simulink model "PubIfDecisionTOS_MDL"  (R2020b)
settings: configuration reference "DspaceConfig" (kept outside this file)
PostLoadFcn:
  | if any(exist('dsrtsu_mdlpostloadfcn', 'file') ~= 0), dsrtsu_mdlpostloadfcn('Execute', bdroot); end
InitFcn:
  | , if any(exist('dsmpb_private', 'file') ~= 0), dsmpb_private('dsmpb_mdlclblib', 'Init', bdroot); end,
undefined symbols (not defined in the file or in its folder): C_TOS_ACCEgoRAxletoFbumplength_m, C_TOS_ACCTargetFront_Flag, C_TOS_AEBJAPedObjDxThre_Val, C_TOS_AEBJAPedObjDyThre_Val, C_TOS_AEBJATargetSize_Val, C_TOS_AEBJAVehObjDxThre_Val, C_TOS_AEBJAVehObjDyThre_Val, C_TOS_AEBJuncPedTargetSize_Val, C_TOS_AEBLatObjDxThre_Val, C_TOS_AEBLatPedDyThre_Val, C_TOS_AEBLatTargetSize_Val, C_TOS_AEBLongTargetInEgoFront_Flag, C_TOS_axAbsGround_Parameter, C_TOS_CameraConfirmedFlag, C_TOS_CNsubjWidth, C_TOS_CurrentLaneCoreMinWidth_Val, C_TOS_CutInProb_Val_Zero, C_TOS_CutOutProb_Val_Zero, C_TOS_D2R_Val, C_TOS_DefaultValueObjectToCenterLine_dy, C_TOS_EgoCarWidth_Val, C_TOS_EgoDxRefPoint_m, C_TOS_EgoRAxletoFbumplength_m, C_TOS_HalfWidthVehicle_Con, C_TOS_HWA_CurrentLaneFlag, C_TOS_HWA_LeftLaneFlag, C_TOS_HWA_MovingDir_Vaild, C_TOS_HWA_MovState_Vaild, C_TOS_HWA_RightLaneFlag, C_TOS_LaneLineCourseErrorFront, C_TOS_LaneLineCourseErrorRear, C_TOS_MotorbikeDefaultWidth_m, C_TOS_NumberOfEffectiveTargets, C_TOS_Obj_Age_Val, C_TOS_Objdx_Constraint_Val, C_TOS_ObjectDefaultWidth_m, C_TOS_ObjInCurrentLane_Val, C_TOS_ObjInCurrentLaneValid, C_TOS_ObjInLeftLaneValid, C_TOS_ObjInRightLaneValid, C_TOS_ObjNotInCurrentLane_Val, C_TOS_ObjNotREElementType, C_TOS_ObjPredictDis_dy_ConstantVal_Zeros, C_TOS_ObjToCenterLine_ConstantVal_Zeros, C_TOS_OFMObjIDInvilad_Val, C_TOS_PIL_LatDisCons_Val_zero, C_TOS_PIL_ObjectCutInFlag_b, C_TOS_PIL_ObjectCutOutFlag_b, C_TOS_PIL_ObjLaneProb_al_Val, C_TOS_PP_ObjFusType_FC_Confirm_b, C_TOS_PP_ObjFusType_FC_FR_Confirm_b, C_TOS_PP_ObjFusType_FR_Confirm_b, C_TOS_RE_80BoolDefault_Val, C_TOS_RE_80Single181Default_Val, C_TOS_RE_80Single255Default_Val, C_TOS_RE_80Uint8Default_Val, C_TOS_RE_D2R, C_TOS_RE_D_180_Val, C_TOS_RE_InvalidObjectID_Val, C_TOS_RE_InvalidTargetChainDir_Val ... (+142)
libraries: simulink x1650, TOS_LIB x361, canfdmsglib x14
(part 12 of 69)

== system PubIfDecisionTOS_MDL/TOS_20201112/TOS_2012080320/TOS/ACC/TOS_ACCLeftLane/ACC_Object_PreConfirm ==
  PP_ObjFusType_FC_FR_Confirm : Inport
  PP_ObjFusType_FR_Confirm : Inport  Port=2
  PP_ObjFusType_FC_Confirm : Inport  Port=3
  Object_ID : Inport  Port=4
  Obj_MovingState : Inport  Port=5
  Obj_Dx : Inport  Port=6
  Object_ObstacleProb : Inport  Port=7
  Object_DY : Inport  Port=8
  Object_Type : Inport  Port=9
  ACC_Target_ID_K1 : Inport  Port=10
  ACC_Target_Dx_K1 : Inport  Port=11
  ACC_Object_PreConfirm : Subsystem
  Bus Creator : BusCreator  Inputs=5
  Unit Delay : UnitDelay  SampleTime=-1  HasFrameUpgradeWarning=on
  Unit Delay1 : UnitDelay  InitialCondition=255  SampleTime=-1  HasFrameUpgradeWarning=on
  TOS_ACC_P2_P4_TargetPreConfirm : Outport
  wires:
  PP_ObjFusType_FR_Confirm/1 -> ACC_Object_PreConfirm/2(PP_ObjFusType_FR_Confirm)
  PP_ObjFusType_FC_FR_Confirm/1 -> ACC_Object_PreConfirm/1(PP_ObjFusType_FC_FR_Confirm)
  PP_ObjFusType_FC_Confirm/1 -> ACC_Object_PreConfirm/3(PP_ObjFusType_FC_Confirm)
  Object_ID/1 -> ACC_Object_PreConfirm/4(Object_ID)
  ACC_Target_Dx_K1/1 -> Unit Delay1/1
  ACC_Target_ID_K1/1 -> Unit Delay/1
  Object_DY/1 -> ACC_Object_PreConfirm/8(Object_DY)
  Object_ObstacleProb/1 -> ACC_Object_PreConfirm/7(Object_ObstacleProb)
  Obj_Dx/1 -> ACC_Object_PreConfirm/6(Obj_Dx)
  Obj_MovingState/1 -> ACC_Object_PreConfirm/5(Obj_MovingState)
  Object_Type/1 -> ACC_Object_PreConfirm/9(Object_ObjType)
  Bus Creator/1 -> TOS_ACC_P2_P4_TargetPreConfirm/1  "TOS_ACC_P2_P4_TargetPre_ObserVale"
  Unit Delay/1 -> ACC_Object_PreConfirm/10(ACC_Target_ID_K1)
  Unit Delay1/1 -> ACC_Object_PreConfirm/11(ACC_Target_Dx_K1)
  ACC_Object_PreConfirm/1(TOS_ACC_TargetPre_Confirm_FiltFlag) -> Bus Creator/1  "TOS_ACC_P2_P4_TargetPre_Confirm_FiltFlag"
  ACC_Object_PreConfirm/2(TOS_ACC_TargetPre_FusionTypeFlag_ObserVale) -> Bus Creator/2  "TOS_ACC_P2_P4_TargetPre_FusionTypeFlag_ObserVale"
  ACC_Object_PreConfirm/3(TOS_ACC_TargetPre_PassedbyTarget_ObserVale) -> Bus Creator/3  "TOS_ACC_P2_P4_TargetPre_PassedbyTarget_ObserVale"
  ACC_Object_PreConfirm/4(TOS_ACC_TargetPre_ObjType_ObserVale) -> Bus Creator/4  "TOS_ACC_P2_P4_TargetPre_ObjType_ObserVale"
  ACC_Object_PreConfirm/5(TOS_ACC_DyConfirm_ObserVale) -> Bus Creator/5  "TOS_ACC_P2_P4_DyConfirm_ObserVale"

== system PubIfDecisionTOS_MDL/TOS_20201112/TOS_2012080320/TOS/ACC/TOS_ACCRightLane/ACCTargetPO35Infor ==
  OFM_SignalVerification : Inport
  TOS_AddAttributes : Inport  Port=2
  TOS_ProbInLaneCalculat : Inport  Port=3
  TOS_ACCPO3TargetIndex : Inport  Port=4  OutDataTypeStr=uint8
  TOS_ACCPO5TargetIndex : Inport  Port=5  OutDataTypeStr=uint8
  Bus Creator : BusCreator  Inputs=3
  Bus Selector : BusSelector  OutputSignals=OFM_SignalVerification,TOS_AddAttributes,TOS_ProbInLaneCalculat
  Bus Selector1 : BusSelector  OutputSignals=OFM_SignalVerification
  TOS_ACCPO3TargetInfor : Stateflow chart  TreatAsAtomicUnit=on
  TOS_ACCPO5TargetInfor : Stateflow chart  TreatAsAtomicUnit=on
  TOS_ACCPO3 : Outport  PortDimensions=1  BusOutputAsStruct=on
  TOS_ACCPO5 : Outport  Port=2
  wires:
  TOS_ACCPO3TargetIndex/1 -> TOS_ACCPO3TargetInfor/4(TOS_ACCPO3TargetIndex)
  Bus Selector/1 -> TOS_ACCPO3TargetInfor/1(OFM_SignalVerification)  "<OFM_SignalVerification>"
  Bus Selector/2 -> TOS_ACCPO3TargetInfor/2(TOS_AddAttributes)  "<TOS_AddAttributes>"
  TOS_AddAttributes/1 -> Bus Creator/2  "TOS_AddAttributes"
  OFM_SignalVerification/1 -> Bus Creator/1  "OFM_SignalVerification"
  Bus Creator/1 -> Bus Selector1/1, Bus Selector/1
  TOS_ProbInLaneCalculat/1 -> Bus Creator/3  "TOS_ProbInLaneCalculat"
  Bus Selector/3 -> TOS_ACCPO3TargetInfor/3(TOS_ProbInLaneCalculat)  "<TOS_ProbInLaneCalculat>"
  TOS_ACCPO3TargetInfor/1(TOS_ACCPO3TargetInfo) -> TOS_ACCPO3/1
  Bus Selector1/1 -> TOS_ACCPO5TargetInfor/1(OFM_SignalVerification)  "<OFM_SignalVerification>"
  TOS_ACCPO5TargetIndex/1 -> TOS_ACCPO5TargetInfor/2(TOS_ACCPO5TargetIndex)
  TOS_ACCPO5TargetInfor/1(TOS_ACCPO5TargetInfo) -> TOS_ACCPO5/1

== system PubIfDecisionTOS_MDL/TOS_20201112/TOS_2012080320/TOS/ACC/TOS_ACCRightLane/ACC_LeftLane_Target ==
  VIE_EgoVelocity : Inport
  OFM_SignalVerification : Inport  Port=2
  TOS_AddAttributes : Inport  Port=3
  TOS_ProbInLaneCalculat : Inport  Port=4
  TOS_VCAN_SignalVerification : Inport  Port=5
  TOS_ACC_P3_P5_Index : Inport  Port=6
  ACC_TargetP3_ID_K1 : Inport  Port=7
  ACC_TargetP3_MovState_K1 : Inport  Port=8
  ACC_TargetP5_ID_K1 : Inport  Port=9
  ACC_TargetP3_ID_K2 : InportShadow  Port=7
  ACC_TargetP3_MovState_K2 : InportShadow  Port=8
  ACC_TargetP5_ID_K2 : InportShadow  Port=9
  ACC_TargetP5_ID_K3 : InportShadow  Port=9
  Bus Creator : BusCreator  Inputs=14
  Bus Creator1 : BusCreator  Inputs=11
  Bus Creator2 : BusCreator  Inputs=11
  Bus Selector : BusSelector  OutputSignals=TOS_ACC_P3_P5_Index,OFM_SignalVerification.Object_ID,OFM_SignalVerification.Object_Fus_Type,OFM_SignalVerification.Object_MovingState,TOS_AddAttributes.PP_ObjMovingDirSignalProcessing,OFM_SignalVerification.Object_HeadingAngle,OFM_SignalVerification.Object_DX,OFM_SignalVerification.Object_Type,OFM_SignalVerification.Object_ObstacleProb,OFM_SignalVerification.Object_DY,TOS_AddAttributes.PP_ObjFusType_FC_FR_Confirm,TOS_AddAttributes.PP_ObjFusType_FR_Confirm,TOS_AddAttributes.PP_ObjFusType_FC_Confirm,OFM_SignalVerification.Object_VX,OFM_SignalVerification.Object_VY,VIE_EgoVelocity,TOS_VCAN_SignalVerification.SteerWheelAng,ACC_TargetP3_ID_K1,ACC_TargetP3_ID_K2,ACC_TargetP3_MovState_K1,ACC_TargetP3_MovState_K2
  Bus Selector1 : BusSelector  OutputSignals=TOS_ACC_P3_P5_Index,OFM_SignalVerification.Object_ID,OFM_SignalVerification.Object_Fus_Type,OFM_SignalVerification.Object_MovingState,TOS_AddAttributes.PP_ObjMovingDirSignalProcessing,OFM_SignalVerification.Object_HeadingAngle,OFM_SignalVerification.Object_DX,OFM_SignalVerification.Object_Type,OFM_SignalVerification.Object_ObstacleProb,OFM_SignalVerification.Object_DY,TOS_AddAttributes.PP_ObjFusType_FC_FR_Confirm,TOS_AddAttributes.PP_ObjFusType_FR_Confirm,TOS_AddAttributes.PP_ObjFusType_FC_Confirm,OFM_SignalVerification.Object_VX,OFM_SignalVerification.Object_VY,VIE_EgoVelocity,TOS_VCAN_SignalVerification.SteerWheelAng,ACC_TargetP5_ID_K1,ACC_TargetP5_ID_K2,ACC_TargetP5_MovState_K1,ACC_TargetP5_MovState_K2
  Bus Selector2 : BusSelector  OutputSignals=PP_MovingStateSignalProcessing
  Data Type Conversion{1..4} (4 alike) : DataTypeConversion  OutDataTypeStr=Enum: ObjectMovingState_E
  Delay{,3..4,7} (4 alike) : Delay  InitialCondition=0
  Delay{1..2,5..6} (4 alike) : Delay  DelayLength=1  InitialCondition=0
  Saturation : Saturate  UpperLimit=uint8(80)  LowerLimit=uint8(1)
  Selector1 : Selector  InputPortWidth=80  IndexOptions=Index vector (port)  Indices=[1 3]  OutputSizes=1
  Selector2 : Selector  InputPortWidth=80  IndexOptions=Index vector (port)  Indices=[1 3]  OutputSizes=1
  TOS_ACC_P3 : Subsystem
  TOS_ACC_P5 : Subsystem
  TOS_AddAttributes1 : InportShadow  Port=3
  Terminator : Terminator
  Terminator1 : Terminator
  TOS_ACC_P3_TragetIndex : Outport
  TOS_ACC_P5_TragetIndex : Outport  Port=2
  wires:
  TOS_AddAttributes/1 -> Bus Creator/3  "TOS_AddAttributes"
  OFM_SignalVerification/1 -> Bus Creator/2
  VIE_EgoVelocity/1 -> Bus Creator/1  "VIE_EgoVelocity"
  TOS_ProbInLaneCalculat/1 -> Bus Creator/4  "TOS_ProbInLaneCalculat"
  TOS_ACC_P3/1(TOS_ACC_P3_Index) -> TOS_ACC_P3_TragetIndex/1  "TOS_ACC_P3_TragetIndex"
  Bus Creator1/1 -> Terminator/1  "TOS_ACC_P3_ObserVale"
  TOS_ACC_P3_P5_Index/1 -> Bus Creator/6  "TOS_ACC_P3_P5_Index"
  TOS_VCAN_SignalVerification/1 -> Bus Creator/5  "TOS_VCAN_SignalVerification"
  Delay1/1 -> Bus Creator/7  "ACC_TargetP3_ID_K1"
  Delay/1 -> Bus Creator/8  "ACC_TargetP3_ID_K2"
  Delay2/1 -> Data Type Conversion2/1
  Data Type Conversion1/1 -> Bus Creator/10  "ACC_TargetP3_MovState_K2"
  ACC_TargetP3_MovState_K2/1 -> Delay3/1
  Data Type Conversion2/1 -> Bus Creator/9  "ACC_TargetP3_MovState_K1"
  Delay3/1 -> Data Type Conversion1/1
  ACC_TargetP3_ID_K2/1 -> Delay/1
  ACC_TargetP3_ID_K1/1 -> Delay1/1
  ACC_TargetP3_MovState_K1/1 -> Delay2/1
  Bus Selector/1 -> TOS_ACC_P3/1(TOS_ACC_P3_P5_Index)  "<TOS_ACC_P3_P5_Index>"
  Bus Selector/2 -> TOS_ACC_P3/2(Object_ID)  "<Object_ID>"
  Bus Selector/3 -> TOS_ACC_P3/3(Object_Fus_Type)  "<Object_Fus_Type>"
  Bus Selector/4 -> TOS_ACC_P3/4(object_MovingState)  "<Object_MovingState>"
  Bus Selector/5 -> TOS_ACC_P3/5(PP_ObjMovingDirSignalProcessing)  "<PP_ObjMovingDirSignalProcessing>"
  Bus Selector/6 -> TOS_ACC_P3/6(Object_HeadingAngle)  "<Object_HeadingAngle>"
  Bus Selector/7 -> TOS_ACC_P3/7(Object_DX)  "<Object_DX>"
  Bus Selector/8 -> TOS_ACC_P3/8(Object_Type)  "<Object_Type>"
  Bus Selector/9 -> TOS_ACC_P3/9(Object_ObstacleProb)  "<Object_ObstacleProb>"
  Bus Selector/10 -> TOS_ACC_P3/10(Object_DY)  "<Object_DY>"
  Bus Selector/11 -> TOS_ACC_P3/11(PP_ObjFusType_FC_FR_Confirm)  "<PP_ObjFusType_FC_FR_Confirm>"
  Bus Selector/12 -> TOS_ACC_P3/12(PP_ObjFusType_FR_Confirm)  "<PP_ObjFusType_FR_Confirm>"
  Bus Selector/13 -> TOS_ACC_P3/13(PP_ObjFusType_FC_Confirm)  "<PP_ObjFusType_FC_Confirm>"
  Bus Selector/14 -> TOS_ACC_P3/14(Object_VX)  "<Object_VX>"
  Bus Selector/15 -> TOS_ACC_P3/15(Object_VY)  "<Object_VY>"
  Bus Selector/16 -> TOS_ACC_P3/16(VIE_EgoVelocity)  "<VIE_EgoVelocity>"
  Bus Selector/17 -> TOS_ACC_P3/17(SteerWheelAng)  "<SteerWheelAng>"
  Bus Selector/18 -> TOS_ACC_P3/18(ACC_TargetP3_ID_K1)  "<ACC_TargetP3_ID_K1>"
  Bus Selector/19 -> TOS_ACC_P3/19(ACC_TargetP3_ID_K2)  "<ACC_TargetP3_ID_K2>"
  Bus Selector/20 -> TOS_ACC_P3/20(ACC_TargetP3_MovState_K1)  "<ACC_TargetP3_MovState_K1>"
  Bus Selector/21 -> TOS_ACC_P3/21(ACC_TargetP3_MovState_K2)  "<ACC_TargetP3_MovState_K2>"
  TOS_ACC_P3/5(TOS_ACC_ObjType_ObserVale) -> Bus Creator1/4  "TOS_ACC_P3_ObjType_ObserVale"
  TOS_ACC_P3/4(TOS_ACC_TargetDxConfirm_ObserVale) -> Bus Creator1/3  "TOS_ACC_P3_TargetDxConfirm_ObserVale"
  TOS_ACC_P3/6(TOS_ACC_ObstacleProb_ObserVale) -> Bus Creator1/5  "TOS_ACC_P3_ObstacleProb_ObserVale"
  TOS_ACC_P3/3(TOS_ACC_TrgMovDir_ObserVale) -> Bus Creator1/2  "TOS_ACC_P3_TrgMovDir_ObserVale"
  TOS_ACC_P3/7(TOS_ACC_TrgMovDirFlag_1_ObserVale) -> Bus Creator1/6  "TOS_ACC_P3_TrgMovDirFlag_1_ObserVale"
  TOS_ACC_P3/2(TOS_ACC_FusionType_ObserVale) -> Bus Creator1/1  "TOS_ACC_P3_FusionType_ObserVale"
  TOS_ACC_P3/8(TOS_ACC_TrgMovDirFlag_2_ObserVale) -> Bus Creator1/7  "TOS_ACC_P3_TrgMovDirFlag_2_ObserVale"
  TOS_ACC_P3/9(TOS_ACC_TrgMovDirFlag_3_ObserVale) -> Bus Creator1/8  "TOS_ACC_P3_TrgMovDirFlag_3_ObserVale"
  TOS_ACC_P3/10(TOS_ACC_TrgMovDirFlag_4_ObserVale) -> Bus Creator1/9  "TOS_ACC_P3_TrgMovDirFlag_4_ObserVale"
  TOS_ACC_P3/11(TOS_ACC_TrgMovDirFlag_5_ObserVale) -> Bus Creator1/10  "TOS_ACC_P3_TrgMovDirFlag_5_ObserVale"
  TOS_ACC_P3/12(TOS_ACC_TrgMovDirFlag_6_ObserVale) -> Bus Creator1/11  "TOS_ACC_P3_TrgMovDirFlag_6_ObserVale"
  Selector1/1 -> Delay6/1
  ACC_TargetP5_ID_K1/1 -> Delay5/1
  ACC_TargetP5_ID_K2/1 -> Delay4/1
  Delay7/1 -> Data Type Conversion4/1
  Data Type Conversion3/1 -> Bus Creator/13  "ACC_TargetP5_MovState_K1"
  Selector2/1 -> Delay7/1
  Data Type Conversion4/1 -> Bus Creator/14  "ACC_TargetP5_MovState_K2"
  Delay6/1 -> Data Type Conversion3/1
  Delay4/1 -> Bus Creator/12  "ACC_TargetP5_ID_K2"
  Delay5/1 -> Bus Creator/11  "ACC_TargetP5_ID_K1"
  Bus Creator/1 -> Bus Selector1/1, Bus Selector/1
  TOS_ACC_P5/12(TOS_ACC_TrgMovDirFlag_6_ObserVale) -> Bus Creator2/11  "TOS_ACC_P5_TrgMovDirFlag_6_ObserVale"
  TOS_ACC_P5/11(TOS_ACC_TrgMovDirFlag_5_ObserVale) -> Bus Creator2/10  "TOS_ACC_P5_TrgMovDirFlag_5_ObserVale"
  TOS_ACC_P5/10(TOS_ACC_TrgMovDirFlag_4_ObserVale) -> Bus Creator2/9  "TOS_ACC_P5_TrgMovDirFlag_4_ObserVale"
  TOS_ACC_P5/9(TOS_ACC_TrgMovDirFlag_3_ObserVale) -> Bus Creator2/8  "TOS_ACC_P5_TrgMovDirFlag_3_ObserVale"
  TOS_ACC_P5/8(TOS_ACC_TrgMovDirFlag_2_ObserVale) -> Bus Creator2/7  "TOS_ACC_P5_TrgMovDirFlag_2_ObserVale"
  TOS_ACC_P5/2(TOS_ACC_FusionType_ObserVale) -> Bus Creator2/1  "TOS_ACC_P5_FusionType_ObserVale"
  TOS_ACC_P5/7(TOS_ACC_TrgMovDirFlag_1_ObserVale) -> Bus Creator2/6  "TOS_ACC_P5_TrgMovDirFlag_1_ObserVale"
  TOS_ACC_P5/3(TOS_ACC_TrgMovDir_ObserVale) -> Bus Creator2/2  "TOS_ACC_P5_TrgMovDir_ObserVale"
  TOS_ACC_P5/6(TOS_ACC_ObstacleProb_ObserVale) -> Bus Creator2/5  "TOS_ACC_P5_ObstacleProb_ObserVale"
  TOS_ACC_P5/4(TOS_ACC_TargetDxConfirm_ObserVale) -> Bus Creator2/3  "TOS_ACC_P5_TargetDxConfirm_ObserVale"
  TOS_ACC_P5/5(TOS_ACC_ObjType_ObserVale) -> Bus Creator2/4  "TOS_ACC_P5_ObjType_ObserVale"
  Bus Selector1/21 -> TOS_ACC_P5/21(ACC_TargetP5_MovState_K2)  "<ACC_TargetP5_MovState_K2>"
  Bus Selector1/20 -> TOS_ACC_P5/20(ACC_TargetP5_MovState_K1)  "<ACC_TargetP5_MovState_K1>"
  Bus Selector1/19 -> TOS_ACC_P5/19(ACC_TargetP5_ID_K2)  "<ACC_TargetP5_ID_K2>"
  Bus Selector1/18 -> TOS_ACC_P5/18(ACC_TargetP5_ID_K1)  "<ACC_TargetP5_ID_K1>"
  Bus Selector1/17 -> TOS_ACC_P5/17(SteerWheelAng)  "<SteerWheelAng>"
  Bus Selector1/16 -> TOS_ACC_P5/16(VIE_EgoVelocity)  "<VIE_EgoVelocity>"
  Bus Selector1/15 -> TOS_ACC_P5/15(Object_VY)  "<Object_VY>"
  Bus Selector1/14 -> TOS_ACC_P5/14(Object_VX)  "<Object_VX>"
  Bus Selector1/13 -> TOS_ACC_P5/13(PP_ObjFusType_FC_Confirm)  "<PP_ObjFusType_FC_Confirm>"
  Bus Selector1/12 -> TOS_ACC_P5/12(PP_ObjFusType_FR_Confirm)  "<PP_ObjFusType_FR_Confirm>"
  Bus Selector1/11 -> TOS_ACC_P5/11(PP_ObjFusType_FC_FR_Confirm)  "<PP_ObjFusType_FC_FR_Confirm>"
  Bus Selector1/10 -> TOS_ACC_P5/10(Object_DY)  "<Object_DY>"
  Bus Selector1/9 -> TOS_ACC_P5/9(Object_ObstacleProb)  "<Object_ObstacleProb>"
  Bus Selector1/8 -> TOS_ACC_P5/8(Object_Type)  "<Object_Type>"
  Bus Selector1/7 -> TOS_ACC_P5/7(Object_DX)  "<Object_DX>"
  Bus Selector1/6 -> TOS_ACC_P5/6(Object_HeadingAngle)  "<Object_HeadingAngle>"
  Bus Selector1/5 -> TOS_ACC_P5/5(PP_ObjMovingDirSignalProcessing)  "<PP_ObjMovingDirSignalProcessing>"
  Bus Selector1/4 -> TOS_ACC_P5/4(object_MovingState)  "<Object_MovingState>"
  Bus Selector1/3 -> TOS_ACC_P5/3(Object_Fus_Type)  "<Object_Fus_Type>"
  Bus Selector1/2 -> TOS_ACC_P5/2(Object_ID)  "<Object_ID>"
  Bus Selector1/1 -> TOS_ACC_P5/1(TOS_ACC_P3_P5_Index)  "<TOS_ACC_P3_P5_Index>"
  Bus Creator2/1 -> Terminator1/1  "TOS_ACC_P5_ObserVale"
  TOS_ACC_P5/1(TOS_ACC_P5_Index) -> TOS_ACC_P5_TragetIndex/1  "TOS_ACC_P5_TragetIndex"
  TOS_AddAttributes1/1 -> Bus Selector2/1  "TOS_AddAttributes"
  Bus Selector2/1 -> Selector1/1, Selector2/1  "<PP_MovingStateSignalProcessing>"
  ACC_TargetP5_ID_K3/1 -> Saturation/1
  Saturation/1 -> Selector1/2, Selector2/2

== system PubIfDecisionTOS_MDL/TOS_20201112/TOS_2012080320/TOS/ACC/TOS_ACCRightLane/ACC_Object_PreConfirm ==
  PP_ObjFusType_FC_FR_Confirm : Inport
  PP_ObjFusType_FR_Confirm : Inport  Port=2
  PP_ObjFusType_FC_Confirm : Inport  Port=3
  Object_ID : Inport  Port=4
  Obj_MovingState : Inport  Port=5
  Obj_Dx : Inport  Port=6
  Object_ObstacleProb : Inport  Port=7
  Object_DY : Inport  Port=8
  Object_Type : Inport  Port=9
  ACC_Target_ID_K1 : Inport  Port=10
  ACC_Target_Dx_K1 : Inport  Port=11
  ACC_Object_PreConfirm : Subsystem
  Bus Creator : BusCreator  Inputs=5
  Unit Delay : UnitDelay  SampleTime=-1  HasFrameUpgradeWarning=on
  Unit Delay1 : UnitDelay  InitialCondition=255  SampleTime=-1  HasFrameUpgradeWarning=on
  TOS_ACC_P3_P5_TargetPreConfirm : Outport
  wires:
  ACC_Object_PreConfirm/5(TOS_ACC_DyConfirm_ObserVale) -> Bus Creator/5  "TOS_ACC_P3_P5_DyConfirm_ObserVale"
  ACC_Object_PreConfirm/4(TOS_ACC_TargetPre_ObjType_ObserVale) -> Bus Creator/4  "TOS_ACC_P3_P5_TargetPre_ObjType_ObserVale"
  ACC_Object_PreConfirm/3(TOS_ACC_TargetPre_PassedbyTarget_ObserVale) -> Bus Creator/3  "TOS_ACC_P3_P5_TargetPre_PassedbyTarget_ObserVale"
  ACC_Object_PreConfirm/2(TOS_ACC_TargetPre_FusionTypeFlag_ObserVale) -> Bus Creator/2  "TOS_ACC_P3_P5_TargetPre_FusionTypeFlag_ObserVale"
  ACC_Object_PreConfirm/1(TOS_ACC_TargetPre_Confirm_FiltFlag) -> Bus Creator/1  "TOS_ACC_P3_P5_TargetPre_Confirm_FiltFlag"
  Unit Delay1/1 -> ACC_Object_PreConfirm/11(ACC_Target_Dx_K1)
  Unit Delay/1 -> ACC_Object_PreConfirm/10(ACC_Target_ID_K1)
  Bus Creator/1 -> TOS_ACC_P3_P5_TargetPreConfirm/1  "TOS_ACC_P3_P5_TargetPre_ObserVale"
  Object_Type/1 -> ACC_Object_PreConfirm/9(Object_ObjType)
  Obj_MovingState/1 -> ACC_Object_PreConfirm/5(Obj_MovingState)
  Obj_Dx/1 -> ACC_Object_PreConfirm/6(Obj_Dx)
  Object_ObstacleProb/1 -> ACC_Object_PreConfirm/7(Object_ObstacleProb)
  Object_DY/1 -> ACC_Object_PreConfirm/8(Object_DY)
  ACC_Target_ID_K1/1 -> Unit Delay/1
  ACC_Target_Dx_K1/1 -> Unit Delay1/1
  Object_ID/1 -> ACC_Object_PreConfirm/4(Object_ID)
  PP_ObjFusType_FC_Confirm/1 -> ACC_Object_PreConfirm/3(PP_ObjFusType_FC_Confirm)
  PP_ObjFusType_FC_FR_Confirm/1 -> ACC_Object_PreConfirm/1(PP_ObjFusType_FC_FR_Confirm)
  PP_ObjFusType_FR_Confirm/1 -> ACC_Object_PreConfirm/2(PP_ObjFusType_FR_Confirm)

== system PubIfDecisionTOS_MDL/TOS_20201112/TOS_2012080320/TOS/AEB/TOS_AEBJunct1105/AEBJuncTargetIndex ==
  TOS_AEBJunc_ConditionPedTargets_Dx : Inport  OutDataTypeStr=single
  TOS_AEBJunc_ConditionPedTargets_Dx1 : Inport  Port=2  OutDataTypeStr=single
  Assignment1 : Assignment  DiagnosticForDimensions=Warning  IndexOptions=Assign all  Indices=1  OutputSizes=1
  Constant1 : Constant  Value=zeros(C_TOS_AEBJATargetSize_Val,1)  OutDataTypeStr=uint8
      settings: AttributesFormatString=%<Value> = 32
  Constant2 : Constant  Value=C_TOS_NumberOfEffectiveTargets  OutDataTypeStr=uint8
      settings: AttributesFormatString=C_TOS_NumberOfEffectiveTargets = 80
  MATLAB Function : MATLAB Function  TreatAsAtomicUnit=on
  MATLAB Function1 : MATLAB Function  TreatAsAtomicUnit=on
  Selector1 : Selector  InputPortWidth=80  IndexOptions=Index vector (dialog)  Indices=1:16  OutputSizes=1
  Selector2 : Selector  InputPortWidth=80  IndexOptions=Index vector (dialog)  Indices=1:16  OutputSizes=1
  Vector Concatenate : Concatenate
  TOS_AEBJuncTargetIndex : Outport
  wires:
  TOS_AEBJunc_ConditionPedTargets_Dx/1 -> MATLAB Function/1(Distance)
  Constant1/1 -> Assignment1/1
  Assignment1/1 -> TOS_AEBJuncTargetIndex/1
  Constant2/1 -> MATLAB Function/2(Object_Num), MATLAB Function1/1(Object_Num)
  MATLAB Function/1(ObjDisIndex) -> Selector1/1  "TOS_AEBJuncPedTargetIndex"
  Selector1/1 -> Vector Concatenate/1
  TOS_AEBJunc_ConditionPedTargets_Dx1/1 -> MATLAB Function1/2(Distance)
  Selector2/1 -> Vector Concatenate/2
  MATLAB Function1/1(ObjDisIndex) -> Selector2/1  "TOS_AEBJuncVehTargetIndex"
  Vector Concatenate/1 -> Assignment1/2

== system PubIfDecisionTOS_MDL/TOS_20201112/TOS_2012080320/TOS/AEB/TOS_AEBJunct1105/AEBJunc_Object_Condition ==
  Object_ID : Inport
  PP_ObjFusType_FC_FR_Confirm : Inport  Port=2
  PP_ObjFusType_FR_Confirm : Inport  Port=3
  ObjectType : Inport  Port=4
  Object_Dx : Inport  Port=5
  Object_Dy : Inport  Port=6
  PP_ObjMovingDirSignalProcessing : Inport  Port=7
  Object_HeadingAngle : Inport  Port=8
  Object_VX : Inport  Port=9
  Object_VY : Inport  Port=10
  VIE_EgoVelocity : Inport  Port=11
  psiDtOpt : Inport  Port=12
  axvRefMs2 : Inport  Port=13
  Object_MovingState : Inport  Port=14
  AEBJunc_Target_ObjectID_K1 : Inport  Port=15
  AEBJunc_Target_ObjectType_K1 : Inport  Port=16
  AEBJA_TargetCondition : Subsystem
  TOS_AEBJunc_PedTargets_Dx : Outport
  TOS_AEBJunc_VehTargets_Dx : Outport  Port=2
  AEBJunc_PedTargetFusionType_observal : Outport  Port=3
  AEBJunc_PedTargetObjectType_observal : Outport  Port=4
  AEBJunc_PedTargetDXDY_observal : Outport  Port=5
  AEBJunc_PedTargetMovDir_observal : Outport  Port=6
  AEBJunc_VehTargetFusionType_observal : Outport  Port=7
  AEBJunc_VehTargetObjectType_observal : Outport  Port=8
  AEBJunc_VehTargetDXDY_observal : Outport  Port=9
  AEBJunc_VehTargetMovDir_observal : Outport  Port=10
  AEBJunc_VehTargetMovState_observal : Outport  Port=11
  wires:
  PP_ObjFusType_FR_Confirm/1 -> AEBJA_TargetCondition/3(PP_ObjFusType_FR_Confirm)
  PP_ObjFusType_FC_FR_Confirm/1 -> AEBJA_TargetCondition/2(PP_ObjFusType_FC_FR_Confirm)
  Object_VY/1 -> AEBJA_TargetCondition/10(Object_VY)
  VIE_EgoVelocity/1 -> AEBJA_TargetCondition/11(VIE_EgoVelocity)
  Object_VX/1 -> AEBJA_TargetCondition/9(Object_VX)
  PP_ObjMovingDirSignalProcessing/1 -> AEBJA_TargetCondition/7(PP_ObjMovingDirSignalProcessing)
  Object_HeadingAngle/1 -> AEBJA_TargetCondition/8(Object_HeadingAngle)
  Object_ID/1 -> AEBJA_TargetCondition/1(Object_ID)
  ObjectType/1 -> AEBJA_TargetCondition/4(ObjectType)
  Object_Dy/1 -> AEBJA_TargetCondition/6(Object_Dy)
  Object_Dx/1 -> AEBJA_TargetCondition/5(Object_Dx)
  AEBJunc_Target_ObjectID_K1/1 -> AEBJA_TargetCondition/15(AEBJunc_Target_ObjectID_K1)
  psiDtOpt/1 -> AEBJA_TargetCondition/12(psiDtOpt)
  axvRefMs2/1 -> AEBJA_TargetCondition/13(axvRefMs2)
  AEBJunc_Target_ObjectType_K1/1 -> AEBJA_TargetCondition/16(AEBJunc_Target_ObjectType_K1)  "AEBJunc_Target_ObjectType_K1"
  AEBJA_TargetCondition/1(TOS_AEBJunc_PedTargets_Dx) -> TOS_AEBJunc_PedTargets_Dx/1
  AEBJA_TargetCondition/7(AEBJunc_VehTargetFusionType_observal) -> AEBJunc_VehTargetFusionType_observal/1
  AEBJA_TargetCondition/8(AEBJunc_VehTargetObjectType_observal) -> AEBJunc_VehTargetObjectType_observal/1
  AEBJA_TargetCondition/9(AEBJunc_VehTargetDXDY_observal) -> AEBJunc_VehTargetDXDY_observal/1
  AEBJA_TargetCondition/10(AEBJunc_VehTargetMovDir_observal) -> AEBJunc_VehTargetMovDir_observal/1
  Object_MovingState/1 -> AEBJA_TargetCondition/14(Object_MovingState)  "Object_MovingState"
  AEBJA_TargetCondition/11(AEBJunc_VehTargetMovState_observal) -> AEBJunc_VehTargetMovState_observal/1
  AEBJA_TargetCondition/2(TOS_AEBJunc_VehTargets_Dx) -> TOS_AEBJunc_VehTargets_Dx/1
  AEBJA_TargetCondition/3(AEBJunc_PedTargetFusionType_observal) -> AEBJunc_PedTargetFusionType_observal/1
  AEBJA_TargetCondition/4(AEBJunc_PedTargetObjectType_observal) -> AEBJunc_PedTargetObjectType_observal/1
  AEBJA_TargetCondition/5(AEBJunc_PedTargetDXDY_observal) -> AEBJunc_PedTargetDXDY_observal/1
  AEBJA_TargetCondition/6(AEBJunc_PedTargetMovDir_observal) -> AEBJunc_PedTargetMovDir_observal/1

== system PubIfDecisionTOS_MDL/TOS_20201112/TOS_2012080320/TOS/AEB/TOS_AEBJunct1105/AEBJunc_Object_Condition1 ==
  Object_ID : Inport
  PP_ObjFusType_FC_FR_Confirm : Inport  Port=2
  PP_ObjFusType_FR_Confirm : Inport  Port=3
  ObjectType : Inport  Port=4
  Object_Dx : Inport  Port=5
  Object_Dy : Inport  Port=6
  PP_ObjMovingDirSignalProcessing : Inport  Port=7
  Object_HeadingAngle : Inport  Port=8
  Object_VX : Inport  Port=9
  Object_VY : Inport  Port=10
  VIE_EgoVelocity : Inport  Port=11
  psiDtOpt : Inport  Port=12
  axvRefMs2 : Inport  Port=13
  Object_MovingState : Inport  Port=14
  AEBJunc_Target_ObjectID_K1 : Inport  Port=15
  AEBJunc_Target_ObjectType_K1 : Inport  Port=16
  AEBJA_TargetCondition : Subsystem
  TOS_AEBJunc_PedTargets_Dx : Outport
  TOS_AEBJunc_VehTargets_Dx : Outport  Port=2
  AEBJunc_PedTargetFusionType_observal : Outport  Port=3
  AEBJunc_PedTargetObjectType_observal : Outport  Port=4
  AEBJunc_PedTargetDXDY_observal : Outport  Port=5
  AEBJunc_PedTargetMovDir_observal : Outport  Port=6
  AEBJunc_VehTargetFusionType_observal : Outport  Port=7
  AEBJunc_VehTargetObjectType_observal : Outport  Port=8
  AEBJunc_VehTargetDXDY_observal : Outport  Port=9
  AEBJunc_VehTargetMovDir_observal : Outport  Port=10
  AEBJunc_VehTargetMovState_observal : Outport  Port=11
  wires:
  AEBJA_TargetCondition/6(AEBJunc_PedTargetMovDir_observal) -> AEBJunc_PedTargetMovDir_observal/1
  AEBJA_TargetCondition/5(AEBJunc_PedTargetDXDY_observal) -> AEBJunc_PedTargetDXDY_observal/1
  AEBJA_TargetCondition/4(AEBJunc_PedTargetObjectType_observal) -> AEBJunc_PedTargetObjectType_observal/1
  AEBJA_TargetCondition/3(AEBJunc_PedTargetFusionType_observal) -> AEBJunc_PedTargetFusionType_observal/1
  AEBJA_TargetCondition/2(TOS_AEBJunc_VehTargets_Dx) -> TOS_AEBJunc_VehTargets_Dx/1
  AEBJA_TargetCondition/11(AEBJunc_VehTargetMovState_observal) -> AEBJunc_VehTargetMovState_observal/1
  Object_MovingState/1 -> AEBJA_TargetCondition/14(Object_MovingState)  "Object_MovingState"
  AEBJA_TargetCondition/10(AEBJunc_VehTargetMovDir_observal) -> AEBJunc_VehTargetMovDir_observal/1
  AEBJA_TargetCondition/9(AEBJunc_VehTargetDXDY_observal) -> AEBJunc_VehTargetDXDY_observal/1
  AEBJA_TargetCondition/8(AEBJunc_VehTargetObjectType_observal) -> AEBJunc_VehTargetObjectType_observal/1
  AEBJA_TargetCondition/7(AEBJunc_VehTargetFusionType_observal) -> AEBJunc_VehTargetFusionType_observal/1
  AEBJA_TargetCondition/1(TOS_AEBJunc_PedTargets_Dx) -> TOS_AEBJunc_PedTargets_Dx/1
  AEBJunc_Target_ObjectType_K1/1 -> AEBJA_TargetCondition/16(AEBJunc_Target_ObjectType_K1)  "AEBJunc_Target_ObjectType_K1"
  axvRefMs2/1 -> AEBJA_TargetCondition/13(axvRefMs2)
  psiDtOpt/1 -> AEBJA_TargetCondition/12(psiDtOpt)
  AEBJunc_Target_ObjectID_K1/1 -> AEBJA_TargetCondition/15(AEBJunc_Target_ObjectID_K1)
  Object_Dx/1 -> AEBJA_TargetCondition/5(Object_Dx)
  Object_Dy/1 -> AEBJA_TargetCondition/6(Object_Dy)
  ObjectType/1 -> AEBJA_TargetCondition/4(ObjectType)
  Object_ID/1 -> AEBJA_TargetCondition/1(Object_ID)
  Object_HeadingAngle/1 -> AEBJA_TargetCondition/8(Object_HeadingAngle)
  PP_ObjMovingDirSignalProcessing/1 -> AEBJA_TargetCondition/7(PP_ObjMovingDirSignalProcessing)
  Object_VX/1 -> AEBJA_TargetCondition/9(Object_VX)
  VIE_EgoVelocity/1 -> AEBJA_TargetCondition/11(VIE_EgoVelocity)
  Object_VY/1 -> AEBJA_TargetCondition/10(Object_VY)
  PP_ObjFusType_FC_FR_Confirm/1 -> AEBJA_TargetCondition/2(PP_ObjFusType_FC_FR_Confirm)
  PP_ObjFusType_FR_Confirm/1 -> AEBJA_TargetCondition/3(PP_ObjFusType_FR_Confirm)

== system PubIfDecisionTOS_MDL/TOS_20201112/TOS_2012080320/TOS/AEB/TOS_AEBJunct1105/AEBJunctionTargetInfor ==
  OFM_SignalVerification : Inport
  TOS_AddAttributes : Inport  Port=2
  TOS_AEBJuncTargetIndex : Inport  Port=3  OutDataTypeStr=uint8
  AEBJunc_Target_ObjectID_K1 : Inport  Port=4
  AEBJunc_Target_ObjectType_K1 : Inport  Port=5
  AEBJuncTargetObjectType : Subsystem
  TOS_AEBJunct : Stateflow chart  TreatAsAtomicUnit=on
  TOS_AEB_JAOBJ : Outport
  wires:
  TOS_AEBJunct/1(TOS_AEBJuncTargetBus) -> TOS_AEB_JAOBJ/1
  TOS_AEBJuncTargetIndex/1 -> TOS_AEBJunct/4(TOS_AEBJATargetIndex), AEBJuncTargetObjectType/4(TOS_AEBJuncTrg_Index)
  OFM_SignalVerification/1 -> AEBJuncTargetObjectType/1(OFM_SignalVerification), TOS_AEBJunct/2(OFM_SignalVerification)
  TOS_AddAttributes/1 -> TOS_AEBJunct/1(TOS_AddAttributes)
  AEBJuncTargetObjectType/1(TOS_AEBJuncTargetObjectType) -> TOS_AEBJunct/3(AEBJuncTargetObjectType)  "AEBJuncTargetObjectType"
  AEBJunc_Target_ObjectID_K1/1 -> AEBJuncTargetObjectType/2(AEBJunc_Target_ObjectID_K1)
  AEBJunc_Target_ObjectType_K1/1 -> AEBJuncTargetObjectType/3(AEBJunc_Target_ObjectType_K1)

== system PubIfDecisionTOS_MDL/TOS_20201112/TOS_2012080320/TOS/AEB/TOS_AEBJunct1105/Subsystem ==
  TOS_AEB_JAOBJ : Inport  Partition=on  PartitionDimension=1  PartitionWidth=1  PartitionOffset=0
  Bus Selector : BusSelector  OutputSignals=ObjectID,ObjectType
  For Each : ForEach  DisableCoverage=on
  ObjectID : Outport  ConcatenationDimension=1
  ObjectType : Outport  Port=2  ConcatenationDimension=1
  wires:
  Bus Selector/1 -> ObjectID/1  "<ObjectID>"
  TOS_AEB_JAOBJ/1 -> Bus Selector/1
  Bus Selector/2 -> ObjectType/1  "<ObjectType>"

== system PubIfDecisionTOS_MDL/TOS_20201112/TOS_2012080320/TOS/AEB/TOS_AEBJunct1105/Subsystem1 ==
  TOS_AEB_JAOBJ : Inport  Partition=on  PartitionDimension=1  PartitionWidth=1  PartitionOffset=0
  Bus Selector : BusSelector  OutputSignals=ObjectID,ObjectType
  For Each : ForEach  DisableCoverage=on
  ObjectID : Outport  ConcatenationDimension=1
  ObjectType : Outport  Port=2  ConcatenationDimension=1
  wires:
  Bus Selector/2 -> ObjectType/1  "<ObjectType>"
  TOS_AEB_JAOBJ/1 -> Bus Selector/1
  Bus Selector/1 -> ObjectID/1  "<ObjectID>"

== system PubIfDecisionTOS_MDL/TOS_20201112/TOS_2012080320/TOS/AEB/TOS_AEBJunct1105/Subsystem2 ==
  TOS_AEB_JAOBJ : Inport  Partition=on  PartitionDimension=1  PartitionWidth=1  PartitionOffset=0
  Bus Selector : BusSelector  OutputSignals=ObjectID,ObjectType
  For Each : ForEach  DisableCoverage=on
  ObjectID : Outport  ConcatenationDimension=1
  ObjectType : Outport  Port=2  ConcatenationDimension=1
  wires:
  Bus Selector/2 -> ObjectType/1  "<ObjectType>"
  TOS_AEB_JAOBJ/1 -> Bus Selector/1
  Bus Selector/1 -> ObjectID/1  "<ObjectID>"

== system PubIfDecisionTOS_MDL/TOS_20201112/TOS_2012080320/TOS/AEB/TOS_AEBJunct1105/TOS_AEBLong_ObserVale ==
  note: Obj_ID
  note: VehMovState
  note: PedMovDir
  note: PedDxDy
  note: PedObjectType
  note: PedFusionType
  note: VehMovDir
  note: VehDxDy
  note: VehFusionType
  note: VehObjectType
  TOS_AEBJunc_TargetIndex : Inport
  TOS_AEBJunc_ObserVale : Inport  Port=2
  Bus Selector3 : BusSelector  OutputSignals=AEBJunc_PedTargetFusionType_observal,AEBJunc_PedTargetObjectType_observal,AEBJunc_PedTargetDXDY_observal,AEBJunc_PedTargetMovDir_observal,AEBJunc_VehTargetFusionType_observal,AEBJunc_VehTargetObjectType_observal,AEBJunc_VehTargetDXDY_observal,AEBJunc_VehTargetMovDir_observal,AEBJunc_VehTargetMovState_observal
  Display{,1..5,23..26} (10 alike) : Display
  wires:
  TOS_AEBJunc_ObserVale/1 -> Bus Selector3/1
  Bus Selector3/1 -> [AEBJunc_PedTargetFusionType_observal]  "<AEBJunc_PedTargetFusionType_observal>"
  Bus Selector3/2 -> [AEBJunc_PedTargetObjectType_observal]  "<AEBJunc_PedTargetObjectType_observal>"
  Bus Selector3/3 -> [TOS_AEBLong_PedTargetDxDy_ObserVale]  "<AEBJunc_PedTargetDXDY_observal>"
  Bus Selector3/4 -> [AEBJunc_PedTargetMovDir_observal]  "<AEBJunc_PedTargetMovDir_observal>"
  Bus Selector3/5 -> [AEBJunc_VehTargetFusionType_observal]  "<AEBJunc_VehTargetFusionType_observal>"
  Bus Selector3/6 -> [AEBJunc_VehTargetObjectType_observal]  "<AEBJunc_VehTargetObjectType_observal>"
  Bus Selector3/7 -> [AEBJunc_VehTargetDxDy_observal]  "<AEBJunc_VehTargetDXDY_observal>"
  Bus Selector3/8 -> [AEBJunc_VehTargetMovDir_observal]  "<AEBJunc_VehTargetMovDir_observal>"
  Bus Selector3/9 -> [AEBJunc_VehTargetMovState_observal]  "<AEBJunc_VehTargetMovState_observal>"
  [AEBJunc_PedTargetFusionType_observal] -> Display26/1
  [AEBJunc_PedTargetObjectType_observal] -> Display25/1
  [TOS_AEBLong_PedTargetDxDy_ObserVale] -> Display24/1
  [AEBJunc_PedTargetMovDir_observal] -> Display23/1
  [AEBJunc_VehTargetFusionType_observal] -> Display/1
  [AEBJunc_VehTargetObjectType_observal] -> Display1/1
  [AEBJunc_VehTargetDxDy_observal] -> Display2/1
  [AEBJunc_VehTargetMovDir_observal] -> Display3/1
  [AEBJunc_VehTargetMovState_observal] -> Display4/1
  TOS_AEBJunc_TargetIndex/1 -> Display5/1

== system PubIfDecisionTOS_MDL/TOS_20201112/TOS_2012080320/TOS/AEB/TOS_AEBJunct_20201208/AEBJuncTargetIndex ==
  TOS_AEBJunc_ConditionPedTargets_Dx : Inport  OutDataTypeStr=single
  TOS_AEBJunc_ConditionPedTargets_Dx1 : Inport  Port=2  OutDataTypeStr=single
  Assignment1 : Assignment  DiagnosticForDimensions=Warning  IndexOptions=Assign all  Indices=1  OutputSizes=1
  Constant1 : Constant  Value=zeros(C_TOS_AEBJATargetSize_Val,1)  OutDataTypeStr=uint8
      settings: AttributesFormatString=%<Value> = 32
  Constant2 : Constant  Value=C_TOS_NumberOfEffectiveTargets  OutDataTypeStr=uint8
      settings: AttributesFormatString=C_TOS_NumberOfEffectiveTargets = 80
  MATLAB Function : MATLAB Function  TreatAsAtomicUnit=on
  MATLAB Function1 : MATLAB Function  TreatAsAtomicUnit=on
  Selector1 : Selector  InputPortWidth=80  IndexOptions=Index vector (dialog)  Indices=1:16  OutputSizes=1
  Selector2 : Selector  InputPortWidth=80  IndexOptions=Index vector (dialog)  Indices=1:16  OutputSizes=1
  Vector Concatenate : Concatenate
  TOS_AEBJuncTargetIndex : Outport
  wires:
  TOS_AEBJunc_ConditionPedTargets_Dx/1 -> MATLAB Function/1(Distance)
  Constant1/1 -> Assignment1/1
  Assignment1/1 -> TOS_AEBJuncTargetIndex/1
  Constant2/1 -> MATLAB Function/2(Object_Num), MATLAB Function1/1(Object_Num)
  MATLAB Function/1(ObjDisIndex) -> Selector1/1  "TOS_AEBJuncPedTargetIndex"
  Selector1/1 -> Vector Concatenate/1
  TOS_AEBJunc_ConditionPedTargets_Dx1/1 -> MATLAB Function1/2(Distance)
  Selector2/1 -> Vector Concatenate/2
  MATLAB Function1/1(ObjDisIndex) -> Selector2/1  "TOS_AEBJuncVehTargetIndex"
  Vector Concatenate/1 -> Assignment1/2

== system PubIfDecisionTOS_MDL/TOS_20201112/TOS_2012080320/TOS/AEB/TOS_AEBJunct_20201208/AEBJunc_Object_Condition ==
  Object_ID : Inport
  PP_ObjFusType_FC_FR_Confirm : Inport  Port=2
  PP_ObjFusType_FR_Confirm : Inport  Port=3
  ObjectType : Inport  Port=4
  Object_Dx : Inport  Port=5
  Object_Dy : Inport  Port=6
  PP_ObjMovingDirSignalProcessing : Inport  Port=7
  Object_HeadingAngle : Inport  Port=8
  Object_VX : Inport  Port=9
  Object_VY : Inport  Port=10
  VIE_EgoVelocity : Inport  Port=11
  psiDtOpt : Inport  Port=12
  axvRefMs2 : Inport  Port=13
  Object_MovingState : Inport  Port=14
  AEBJunc_Target_ObjectID_K1 : Inport  Port=15
  AEBJunc_Target_ObjectType_K1 : Inport  Port=16
  AEBJA_TargetCondition : Subsystem
  TOS_AEBJunc_PedTargets_Dx : Outport
  TOS_AEBJunc_VehTargets_Dx : Outport  Port=2
  AEBJunc_PedTargetFusionType_observal : Outport  Port=3
  AEBJunc_PedTargetObjectType_observal : Outport  Port=4
  AEBJunc_PedTargetDXDY_observal : Outport  Port=5
  AEBJunc_PedTargetMovDir_observal : Outport  Port=6
  AEBJunc_VehTargetFusionType_observal : Outport  Port=7
  AEBJunc_VehTargetObjectType_observal : Outport  Port=8
  AEBJunc_VehTargetDXDY_observal : Outport  Port=9
  AEBJunc_VehTargetMovDir_observal : Outport  Port=10
  AEBJunc_VehTargetMovState_observal : Outport  Port=11
  wires:
  PP_ObjFusType_FR_Confirm/1 -> AEBJA_TargetCondition/3(PP_ObjFusType_FR_Confirm)
  PP_ObjFusType_FC_FR_Confirm/1 -> AEBJA_TargetCondition/2(PP_ObjFusType_FC_FR_Confirm)
  Object_VY/1 -> AEBJA_TargetCondition/10(Object_VY)
  VIE_EgoVelocity/1 -> AEBJA_TargetCondition/11(VIE_EgoVelocity)
  Object_VX/1 -> AEBJA_TargetCondition/9(Object_VX)
  PP_ObjMovingDirSignalProcessing/1 -> AEBJA_TargetCondition/7(PP_ObjMovingDirSignalProcessing)
  Object_HeadingAngle/1 -> AEBJA_TargetCondition/8(Object_HeadingAngle)
  Object_ID/1 -> AEBJA_TargetCondition/1(Object_ID)
  ObjectType/1 -> AEBJA_TargetCondition/4(ObjectType)
  Object_Dy/1 -> AEBJA_TargetCondition/6(Object_Dy)
  Object_Dx/1 -> AEBJA_TargetCondition/5(Object_Dx)
  AEBJunc_Target_ObjectID_K1/1 -> AEBJA_TargetCondition/15(AEBJunc_Target_ObjectID_K1)
  psiDtOpt/1 -> AEBJA_TargetCondition/12(psiDtOpt)
  axvRefMs2/1 -> AEBJA_TargetCondition/13(axvRefMs2)
  AEBJunc_Target_ObjectType_K1/1 -> AEBJA_TargetCondition/16(AEBJunc_Target_ObjectType_K1)  "AEBJunc_Target_ObjectType_K1"
  AEBJA_TargetCondition/1(TOS_AEBJunc_PedTargets_Dx) -> TOS_AEBJunc_PedTargets_Dx/1
  AEBJA_TargetCondition/7(AEBJunc_VehTargetFusionType_observal) -> AEBJunc_VehTargetFusionType_observal/1
  AEBJA_TargetCondition/8(AEBJunc_VehTargetObjectType_observal) -> AEBJunc_VehTargetObjectType_observal/1
  AEBJA_TargetCondition/9(AEBJunc_VehTargetDXDY_observal) -> AEBJunc_VehTargetDXDY_observal/1
  AEBJA_TargetCondition/10(AEBJunc_VehTargetMovDir_observal) -> AEBJunc_VehTargetMovDir_observal/1
  Object_MovingState/1 -> AEBJA_TargetCondition/14(Object_MovingState)  "Object_MovingState"
  AEBJA_TargetCondition/11(AEBJunc_VehTargetMovState_observal) -> AEBJunc_VehTargetMovState_observal/1
  AEBJA_TargetCondition/2(TOS_AEBJunc_VehTargets_Dx) -> TOS_AEBJunc_VehTargets_Dx/1
  AEBJA_TargetCondition/3(AEBJunc_PedTargetFusionType_observal) -> AEBJunc_PedTargetFusionType_observal/1
  AEBJA_TargetCondition/4(AEBJunc_PedTargetObjectType_observal) -> AEBJunc_PedTargetObjectType_observal/1
  AEBJA_TargetCondition/5(AEBJunc_PedTargetDXDY_observal) -> AEBJunc_PedTargetDXDY_observal/1
  AEBJA_TargetCondition/6(AEBJunc_PedTargetMovDir_observal) -> AEBJunc_PedTargetMovDir_observal/1

== system PubIfDecisionTOS_MDL/TOS_20201112/TOS_2012080320/TOS/AEB/TOS_AEBJunct_20201208/AEBJunc_Object_Condition1 ==
  Object_ID : Inport
  PP_ObjFusType_FC_FR_Confirm : Inport  Port=2
  PP_ObjFusType_FR_Confirm : Inport  Port=3
  ObjectType : Inport  Port=4
  Object_Dx : Inport  Port=5
  Object_Dy : Inport  Port=6
  PP_ObjMovingDirSignalProcessing : Inport  Port=7
  Object_HeadingAngle : Inport  Port=8
  Object_VX : Inport  Port=9
  Object_VY : Inport  Port=10
  VIE_EgoVelocity : Inport  Port=11
  psiDtOpt : Inport  Port=12
  axvRefMs2 : Inport  Port=13
  Object_MovingState : Inport  Port=14
  AEBJunc_Target_ObjectID_K1 : Inport  Port=15
  AEBJunc_Target_ObjectType_K1 : Inport  Port=16
  AEBJA_TargetCondition : Subsystem
  TOS_AEBJunc_PedTargets_Dx : Outport
  TOS_AEBJunc_VehTargets_Dx : Outport  Port=2
  AEBJunc_PedTargetFusionType_observal : Outport  Port=3
  AEBJunc_PedTargetObjectType_observal : Outport  Port=4
  AEBJunc_PedTargetDXDY_observal : Outport  Port=5
  AEBJunc_PedTargetMovDir_observal : Outport  Port=6
  AEBJunc_VehTargetFusionType_observal : Outport  Port=7
  AEBJunc_VehTargetObjectType_observal : Outport  Port=8
  AEBJunc_VehTargetDXDY_observal : Outport  Port=9
  AEBJunc_VehTargetMovDir_observal : Outport  Port=10
  AEBJunc_VehTargetMovState_observal : Outport  Port=11
  wires:
  AEBJA_TargetCondition/6(AEBJunc_PedTargetMovDir_observal) -> AEBJunc_PedTargetMovDir_observal/1
  AEBJA_TargetCondition/5(AEBJunc_PedTargetDXDY_observal) -> AEBJunc_PedTargetDXDY_observal/1
  AEBJA_TargetCondition/4(AEBJunc_PedTargetObjectType_observal) -> AEBJunc_PedTargetObjectType_observal/1
  AEBJA_TargetCondition/3(AEBJunc_PedTargetFusionType_observal) -> AEBJunc_PedTargetFusionType_observal/1
  AEBJA_TargetCondition/2(TOS_AEBJunc_VehTargets_Dx) -> TOS_AEBJunc_VehTargets_Dx/1
  AEBJA_TargetCondition/11(AEBJunc_VehTargetMovState_observal) -> AEBJunc_VehTargetMovState_observal/1
  Object_MovingState/1 -> AEBJA_TargetCondition/14(Object_MovingState)  "Object_MovingState"
  AEBJA_TargetCondition/10(AEBJunc_VehTargetMovDir_observal) -> AEBJunc_VehTargetMovDir_observal/1
  AEBJA_TargetCondition/9(AEBJunc_VehTargetDXDY_observal) -> AEBJunc_VehTargetDXDY_observal/1
  AEBJA_TargetCondition/8(AEBJunc_VehTargetObjectType_observal) -> AEBJunc_VehTargetObjectType_observal/1
  AEBJA_TargetCondition/7(AEBJunc_VehTargetFusionType_observal) -> AEBJunc_VehTargetFusionType_observal/1
  AEBJA_TargetCondition/1(TOS_AEBJunc_PedTargets_Dx) -> TOS_AEBJunc_PedTargets_Dx/1
  AEBJunc_Target_ObjectType_K1/1 -> AEBJA_TargetCondition/16(AEBJunc_Target_ObjectType_K1)  "AEBJunc_Target_ObjectType_K1"
  axvRefMs2/1 -> AEBJA_TargetCondition/13(axvRefMs2)
  psiDtOpt/1 -> AEBJA_TargetCondition/12(psiDtOpt)
  AEBJunc_Target_ObjectID_K1/1 -> AEBJA_TargetCondition/15(AEBJunc_Target_ObjectID_K1)
  Object_Dx/1 -> AEBJA_TargetCondition/5(Object_Dx)
  Object_Dy/1 -> AEBJA_TargetCondition/6(Object_Dy)
  ObjectType/1 -> AEBJA_TargetCondition/4(ObjectType)
  Object_ID/1 -> AEBJA_TargetCondition/1(Object_ID)
  Object_HeadingAngle/1 -> AEBJA_TargetCondition/8(Object_HeadingAngle)
  PP_ObjMovingDirSignalProcessing/1 -> AEBJA_TargetCondition/7(PP_ObjMovingDirSignalProcessing)
  Object_VX/1 -> AEBJA_TargetCondition/9(Object_VX)
  VIE_EgoVelocity/1 -> AEBJA_TargetCondition/11(VIE_EgoVelocity)
  Object_VY/1 -> AEBJA_TargetCondition/10(Object_VY)
  PP_ObjFusType_FC_FR_Confirm/1 -> AEBJA_TargetCondition/2(PP_ObjFusType_FC_FR_Confirm)
  PP_ObjFusType_FR_Confirm/1 -> AEBJA_TargetCondition/3(PP_ObjFusType_FR_Confirm)

== system PubIfDecisionTOS_MDL/TOS_20201112/TOS_2012080320/TOS/AEB/TOS_AEBJunct_20201208/AEBJunctionTargetInfor ==
  OFM_SignalVerification : Inport
  TOS_AddAttributes : Inport  Port=2
  TOS_AEBJuncTargetIndex : Inport  Port=3  OutDataTypeStr=uint8
  AEBJunc_Target_ObjectID_K1 : Inport  Port=4
  AEBJunc_Target_ObjectType_K1 : Inport  Port=5
  AEBJuncTargetObjectType : Subsystem
  TOS_AEBJunct : Stateflow chart  TreatAsAtomicUnit=on
  TOS_AEB_JAOBJ : Outport
  wires:
  TOS_AEBJunct/1(TOS_AEBJuncTargetBus) -> TOS_AEB_JAOBJ/1
  TOS_AEBJuncTargetIndex/1 -> TOS_AEBJunct/4(TOS_AEBJATargetIndex), AEBJuncTargetObjectType/4(TOS_AEBJuncTrg_Index)
  OFM_SignalVerification/1 -> AEBJuncTargetObjectType/1(OFM_SignalVerification), TOS_AEBJunct/2(OFM_SignalVerification)
  TOS_AddAttributes/1 -> TOS_AEBJunct/1(TOS_AddAttributes)
  AEBJuncTargetObjectType/1(TOS_AEBJuncTargetObjectType) -> TOS_AEBJunct/3(AEBJuncTargetObjectType)  "AEBJuncTargetObjectType"
  AEBJunc_Target_ObjectID_K1/1 -> AEBJuncTargetObjectType/2(AEBJunc_Target_ObjectID_K1)
  AEBJunc_Target_ObjectType_K1/1 -> AEBJuncTargetObjectType/3(AEBJunc_Target_ObjectType_K1)

== system PubIfDecisionTOS_MDL/TOS_20201112/TOS_2012080320/TOS/AEB/TOS_AEBJunct_20201208/Subsystem ==
  TOS_AEB_JAOBJ : Inport  Partition=on  PartitionDimension=1  PartitionWidth=1  PartitionOffset=0
  Bus Selector : BusSelector  OutputSignals=ObjectID,ObjectType
  For Each : ForEach  DisableCoverage=on
  ObjectID : Outport  ConcatenationDimension=1
  ObjectType : Outport  Port=2  ConcatenationDimension=1
  wires:
  Bus Selector/1 -> ObjectID/1  "<ObjectID>"
  TOS_AEB_JAOBJ/1 -> Bus Selector/1
  Bus Selector/2 -> ObjectType/1  "<ObjectType>"

== system PubIfDecisionTOS_MDL/TOS_20201112/TOS_2012080320/TOS/AEB/TOS_AEBJunct_20201208/Subsystem1 ==
  TOS_AEB_JAOBJ : Inport  Partition=on  PartitionDimension=1  PartitionWidth=1  PartitionOffset=0
  Bus Selector : BusSelector  OutputSignals=ObjectID,ObjectType
  For Each : ForEach  DisableCoverage=on
  ObjectID : Outport  ConcatenationDimension=1
  ObjectType : Outport  Port=2  ConcatenationDimension=1
  wires:
  Bus Selector/2 -> ObjectType/1  "<ObjectType>"
  TOS_AEB_JAOBJ/1 -> Bus Selector/1
  Bus Selector/1 -> ObjectID/1  "<ObjectID>"

== system PubIfDecisionTOS_MDL/TOS_20201112/TOS_2012080320/TOS/AEB/TOS_AEBJunct_20201208/Subsystem2 ==
  TOS_AEB_JAOBJ : Inport  Partition=on  PartitionDimension=1  PartitionWidth=1  PartitionOffset=0
  Bus Selector : BusSelector  OutputSignals=ObjectID,ObjectType
  For Each : ForEach  DisableCoverage=on
  ObjectID : Outport  ConcatenationDimension=1
  ObjectType : Outport  Port=2  ConcatenationDimension=1
  wires:
  Bus Selector/2 -> ObjectType/1  "<ObjectType>"
  TOS_AEB_JAOBJ/1 -> Bus Selector/1
  Bus Selector/1 -> ObjectID/1  "<ObjectID>"

== system PubIfDecisionTOS_MDL/TOS_20201112/TOS_2012080320/TOS/AEB/TOS_AEBJunct_20201208/TOS_AEBLong_ObserVale ==
  note: Obj_ID
  note: VehMovState
  note: PedMovDir
  note: PedDxDy
  note: PedObjectType
  note: PedFusionType
  note: VehMovDir
  note: VehDxDy
  note: VehFusionType
  note: VehObjectType
  TOS_AEBJunc_TargetIndex : Inport
  TOS_AEBJunc_ObserVale : Inport  Port=2
  Bus Selector3 : BusSelector  OutputSignals=AEBJunc_PedTargetFusionType_observal,AEBJunc_PedTargetObjectType_observal,AEBJunc_PedTargetDXDY_observal,AEBJunc_PedTargetMovDir_observal,AEBJunc_VehTargetFusionType_observal,AEBJunc_VehTargetObjectType_observal,AEBJunc_VehTargetDXDY_observal,AEBJunc_VehTargetMovDir_observal,AEBJunc_VehTargetMovState_observal
  Display{,1..5,23..26} (10 alike) : Display
  wires:
  TOS_AEBJunc_ObserVale/1 -> Bus Selector3/1
  Bus Selector3/1 -> [AEBJunc_PedTargetFusionType_observal]  "<AEBJunc_PedTargetFusionType_observal>"
  Bus Selector3/2 -> [AEBJunc_PedTargetObjectType_observal]  "<AEBJunc_PedTargetObjectType_observal>"
  Bus Selector3/3 -> [TOS_AEBLong_PedTargetDxDy_ObserVale]  "<AEBJunc_PedTargetDXDY_observal>"
  Bus Selector3/4 -> [AEBJunc_PedTargetMovDir_observal]  "<AEBJunc_PedTargetMovDir_observal>"
  Bus Selector3/5 -> [AEBJunc_VehTargetFusionType_observal]  "<AEBJunc_VehTargetFusionType_observal>"
  Bus Selector3/6 -> [AEBJunc_VehTargetObjectType_observal]  "<AEBJunc_VehTargetObjectType_observal>"
  Bus Selector3/7 -> [AEBJunc_VehTargetDxDy_observal]  "<AEBJunc_VehTargetDXDY_observal>"
  Bus Selector3/8 -> [AEBJunc_VehTargetMovDir_observal]  "<AEBJunc_VehTargetMovDir_observal>"
  Bus Selector3/9 -> [AEBJunc_VehTargetMovState_observal]  "<AEBJunc_VehTargetMovState_observal>"
  [AEBJunc_PedTargetFusionType_observal] -> Display26/1
  [AEBJunc_PedTargetObjectType_observal] -> Display25/1
  [TOS_AEBLong_PedTargetDxDy_ObserVale] -> Display24/1
  [AEBJunc_PedTargetMovDir_observal] -> Display23/1
  [AEBJunc_VehTargetFusionType_observal] -> Display/1
  [AEBJunc_VehTargetObjectType_observal] -> Display1/1
  [AEBJunc_VehTargetDxDy_observal] -> Display2/1
  [AEBJunc_VehTargetMovDir_observal] -> Display3/1
  [AEBJunc_VehTargetMovState_observal] -> Display4/1
  TOS_AEBJunc_TargetIndex/1 -> Display5/1

== system PubIfDecisionTOS_MDL/TOS_20201112/TOS_2012080320/TOS/AEB/TOS_AEBLatCro1105/AEBLatTrgInfor ==
  OFM_SignalVerification : Inport
  TOS_AddAttributes : Inport  Port=2
  TOS_AEBLatTrg_Index : Inport  Port=3  OutDataTypeStr=uint8
  AEBLat_Target_ObjectID_K1 : Inport  Port=4
  AEBLat_Target_ObjectType_K1 : Inport  Port=5
  AEBLatTargetObjectType : Subsystem
  TOS_AEBLatCro : Stateflow chart  TreatAsAtomicUnit=on
  TOS_AEB_LATOBJ : Outport
  wires:
  TOS_AddAttributes/1 -> TOS_AEBLatCro/1(TOS_AddAttributes)
  TOS_AEBLatTrg_Index/1 -> AEBLatTargetObjectType/4(TOS_AEBLatTrg_Index), TOS_AEBLatCro/4(TOS_AEBLatTargetIndex)
  TOS_AEBLatCro/1(TOS_AEBLatTargetBus) -> TOS_AEB_LATOBJ/1
  OFM_SignalVerification/1 -> AEBLatTargetObjectType/1(OFM_SignalVerification), TOS_AEBLatCro/2(OFM_SignalVerification)
  AEBLatTargetObjectType/1(TOS_AEBLatTargetObjectType) -> TOS_AEBLatCro/3(AEBLat_TargetObjectType)  "AEBLat_TargetObjectType"
  AEBLat_Target_ObjectID_K1/1 -> AEBLatTargetObjectType/2(AEBLat_Target_ObjectID_K1)
  AEBLat_Target_ObjectType_K1/1 -> AEBLatTargetObjectType/3(AEBLat_Target_ObjectType_K1)

== system PubIfDecisionTOS_MDL/TOS_20201112/TOS_2012080320/TOS/AEB/TOS_AEBLatCro1105/AEBLat_Object_Condition ==
  Object_ID : Inport
  PP_ObjFusType_FC_FR_Confirm : Inport  Port=2
  PP_ObjFusType_FR_Confirm : Inport  Port=3
  ObjectType : Inport  Port=4
  Object_Dx : Inport  Port=5
  Object_Dy : Inport  Port=6
  PP_ObjMovingDirSignalProcessing : Inport  Port=7
  Object_HeadingAngle : Inport  Port=8
  Object_VX : Inport  Port=9
  Object_VY : Inport  Port=10
  VIE_EgoVelocity : Inport  Port=11
  psiDtOpt : Inport  Port=12
  AEBLat_Target_ObjectID_K1 : Inport  Port=13
  AEBLat_Target_ObjectType_K1 : Inport  Port=14
  AEBLat_TargetCondition : Subsystem
  Terminator : Terminator
  TOS_AEBLat_ConditionTargets_Dx : Outport
  AEBLat_TargetFusionType_observal : Outport  Port=2
  AEBLat_TargetObjectType_observal : Outport  Port=3
  AEBLat_TargetDXDY_observal : Outport  Port=4
  AEBLat_TargetMovDir_observal : Outport  Port=5
  wires:
  PP_ObjFusType_FR_Confirm/1 -> AEBLat_TargetCondition/3(PP_ObjFusType_FR_Confirm)
  PP_ObjFusType_FC_FR_Confirm/1 -> AEBLat_TargetCondition/2(PP_ObjFusType_FC_FR_Confirm)
  Object_VY/1 -> AEBLat_TargetCondition/10(Object_VY)
  VIE_EgoVelocity/1 -> AEBLat_TargetCondition/11(VIE_EgoVelocity)
  Object_VX/1 -> AEBLat_TargetCondition/9(Object_VX)
  PP_ObjMovingDirSignalProcessing/1 -> AEBLat_TargetCondition/7(PP_ObjMovingDirSignalProcessing)
  Object_HeadingAngle/1 -> AEBLat_TargetCondition/8(Object_HeadingAngle)
  Object_ID/1 -> AEBLat_TargetCondition/1(Object_ID)
  ObjectType/1 -> AEBLat_TargetCondition/4(ObjectType)
  Object_Dy/1 -> AEBLat_TargetCondition/6(Object_Dy)
  Object_Dx/1 -> AEBLat_TargetCondition/5(Object_Dx)
  AEBLat_TargetCondition/1(TOS_AEBLat_Targets_Dx) -> TOS_AEBLat_ConditionTargets_Dx/1
  AEBLat_TargetCondition/2(AEBLat_TargetFusionType_observal) -> AEBLat_TargetFusionType_observal/1
  AEBLat_TargetCondition/3(AEBLat_TargetObjectType_observal) -> AEBLat_TargetObjectType_observal/1
  AEBLat_TargetCondition/4(AEBLat_TargetDXDY_observal) -> AEBLat_TargetDXDY_observal/1
  AEBLat_TargetCondition/5(AEBLat_TargetMovDir_observal) -> AEBLat_TargetMovDir_observal/1
  AEBLat_Target_ObjectID_K1/1 -> AEBLat_TargetCondition/13(AEBLat_Target_ObjectID_K1)
  psiDtOpt/1 -> AEBLat_TargetCondition/12(psiDtOpt)
  AEBLat_Target_ObjectType_K1/1 -> Terminator/1
